simulink model "ChargeMgmt"  (R2023a)
settings: configuration reference "AutosarConfig" (kept outside this file)
values from neighbouring files (symbols this model uses):
  currentFactor = 20.0    [BMS_Software_DD.sldd]
  CV_Gain = 0.5    [BMS_Software_DD.sldd]
  MaxCellVoltThrsld = 4.15    [BMS_Software_DD.sldd]
  MaxChrgCurrLimit = 3.3    [BMS_Software_DD.sldd]
  noCurrent = 0.0    [BMS_Software_DD.sldd]
  voltThreshold = 4.1    [BMS_Software_DD.sldd]
undefined symbols (not defined in the file or in its folder): Np_Module
settings Model: DataDictionary=BMS_Software_DD.sldd  EnableAccessToBaseWorkspace=off  Creator=cpatel  LastModifiedBy=cpatel
settings ConfigSetRef: SourceName=AutosarConfig

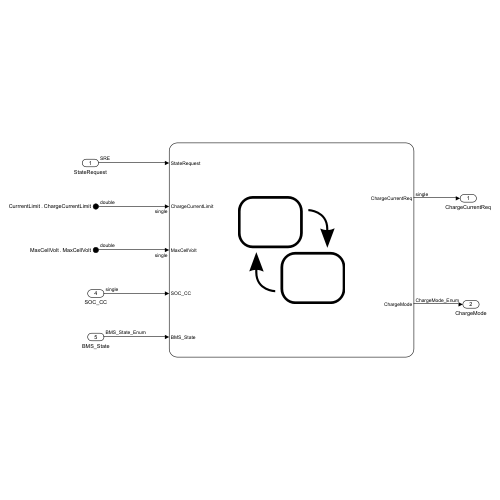
[thumbnail: Simulink's stored preview of the top-level diagram]
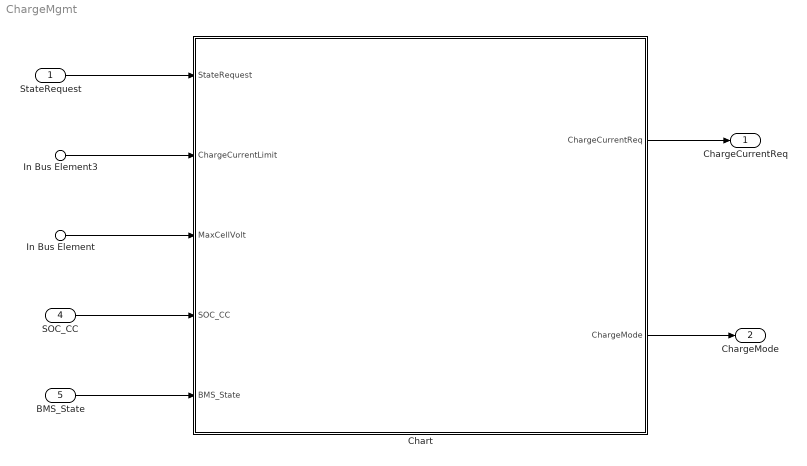
== system ChargeMgmt ==
  StateRequest : Inport  OutDataTypeStr=Enum: SRE  PortDimensions=1
  In Bus Element3 : Inport  Port=2  PortName=CurrrentLimit  Element=ChargeCurrentLimit
  In Bus Element : Inport  Port=3  PortName=MaxCellVolt  Element=MaxCellVolt
  SOC_CC : Inport  Port=4
  BMS_State : Inport  Port=5  OutDataTypeStr=Enum: BMS_State_Enum
  Chart : Stateflow chart  TreatAsAtomicUnit=on
  ChargeCurrentReq : Outport
  ChargeMode : Outport  Port=2
  wires:
  In Bus Element3/1 -> Chart/2(ChargeCurrentLimit)
  In Bus Element/1 -> Chart/3(MaxCellVolt)
  SOC_CC/1 -> Chart/4(SOC_CC)
  BMS_State/1 -> Chart/5(BMS_State)
  StateRequest/1 -> Chart/1(StateRequest)
  Chart/1(ChargeCurrentReq) -> ChargeCurrentReq/1
  Chart/2(ChargeMode) -> ChargeMode/1

== stateflow chart ChargeMgmt/Chart ==
  state ChrgStandby
    en:
    ChargeMode = ChargeMode_Enum.ChrgStandby;
    ChargeCurrentReq = noCurrent;
  state ChrgCC
    en:
    ChargeMode = ChargeMode_Enum.CC;
    du:
    ChargeCurrentReq = ChargeCurrentLimit;
  state ChrgCV
    en:
    ChargeMode = ChargeMode_Enum.CV;
    du:
    ChargeCurrentReq = ChargeCurrentReq - CV_Gain*(MaxCellVolt - MaxCellVoltThrsld);
    ChargeCurrentReq = min(ChargeCurrentReq, ChargeCurrentLimit);
  (default) -> ChrgStandby
  ChrgCV -> ChrgStandby : [StateRequest ~= SRE.Charging || ...
      | ChargeCurrentReq <= (MaxChrgCurrLimit*Np_Module/currentFactor) || ...
      | max(SOC_CC) >single(0.98)]
  ChrgCC -> ChrgStandby [order 1] : [StateRequest ~= SRE.Charging]
  ChrgStandby -> ChrgCC : [StateRequest == SRE.Charging && ...
      | BMS_State == BMS_State_Enum.BMS_Charging && ...
      | MaxCellVolt < voltThreshold && ...
      | max(SOC_CC) < single(0.95)]
  ChrgCC -> ChrgCV [order 2] : [MaxCellVolt>=...
      | MaxCellVoltThrsld]
  data: StateRequest input; ChargeCurrentLimit input; MaxCellVolt input; SOC_CC input; ChargeCurrentReq output; CV_Gain parameter; voltThreshold parameter; noCurrent parameter; MaxCellVoltThrsld parameter; Np_Module parameter; currentFactor parameter; MaxChrgCurrLimit parameter; ChargeMode output; BMS_State input
